simulink model "TPF_Control_Automatico_SLX"  (R2021a)
settings: Solver=ode4  StartTime=0.0  StopTime=30  FixedStep=1e-3  RelTol=1e-3
PreLoadFcn:
  | cuentas_pendulo_doble_final;
InitFcn:
  | cuentas_pendulo_doble_final;
values from neighbouring files (symbols this model uses):
  I0 = 0    [TPF_Control_Automatico.m]    (also in cuentas_pendulo_doble_final.m)
  I1 = m1_value*(((L1_value)^2)/12)    (= 0.0833333333333)    [TPF_Control_Automatico.m]    (also in cuentas_pendulo_doble_final.m; cuentas_prueba.m = 0.0104166666667)
  I2 = m2_value*(((L2_value)^2)/12)    (= 0.1875)    [TPF_Control_Automatico.m]    (also in cuentas_pendulo_doble_final.m; cuentas_prueba.m = 0.03515625)
  K = place(sys.A, sys.B, [-3 -2.5 -2.4 -2 -1.9 -1.8])    [TPF_Control_Automatico.m]    (also in cuentas_pendulo_doble.m = acker(A,B,[0.002,-0.001,-0.001,-0.001,-0.001,-0.001]); cuentas_pendulo_doble_final.m = place(sys.A, sys.B, [-4 -3.5 -3 -2.5 -2 -1.5]); cuentas_prueba.m = acker(sys.A, sys.B, [-3 -3 -2 -2]))
  KDisc = place(sysDisc.A, sysDisc.B, exp([-1.5 -1.6 -1.7 -2 -2.1 -2.2].*Ts))    [TPF_Control_Automatico.m]    (also in cuentas_pendulo_doble_final.m = place(sysDisc.A, sysDisc.B, exp([-3.5 -3 -2.5 -2 -1.5 -1].*T; cuentas_prueba.m = acker(sysDisc.A, sysDisc.B, exp([-2 -2 -1 -1].*Ts)))
  L = place((sys.A)',(sys.C)', [-3 -2.5 -2.4 -2 -1.9 -1.8].*10)'    [TPF_Control_Automatico.m]    (also in cuentas_pendulo_doble.m = [zeros(3,1); cuentas_pendulo_doble_final.m = place((sys.A)',(sys.C)', [-4 -3.5 -3 -2.5 -2 -1.5].*15)'; cuentas_prueba.m = place((sys.A)',(sys.C)', [-25 -20 -35 -30])')
  L1_value = 1    [TPF_Control_Automatico.m]    (also in cuentas_pendulo_doble.m = 0.5; cuentas_pendulo_doble_final.m; cuentas_prueba.m = 0.5)
  L2_value = 1.5    [TPF_Control_Automatico.m]    (also in cuentas_pendulo_doble.m = 0.75; cuentas_pendulo_doble_final.m; cuentas_prueba.m = 0.75)
  LDisc = place((sysDisc.A)',(sysDisc.C)', exp(([-1.5 -1.6 -1.7 -2 -2.1 -2.2].*20).*Ts))'    [TPF_Control_Automatico.m]    (also in cuentas_pendulo_doble_final.m = place((sysDisc.A)',(sysDisc.C)', exp(([-3.5 -3 -2.5 -2 -1.5 ; cuentas_prueba.m = place((sysDisc.A)',(sysDisc.C)', exp([-20 -15 -25 -30].*Ts)))
  m0_value = 5    [TPF_Control_Automatico.m]    (also in cuentas_pendulo_doble.m = 1.5; cuentas_pendulo_doble_final.m; cuentas_prueba.m = 1.5)
  m1_value = 1    [TPF_Control_Automatico.m]    (also in cuentas_pendulo_doble.m = 0.5; cuentas_pendulo_doble_final.m; cuentas_prueba.m = 0.5)
  m2_value = 1    [TPF_Control_Automatico.m]    (also in cuentas_pendulo_doble.m = 0.75; cuentas_pendulo_doble_final.m; cuentas_prueba.m = 0.75)
  s = tf('s')    [TPF_Control_Automatico.m]    (also in cuentas_pendulo_doble.m; cuentas_pendulo_doble_final.m; cuentas_prueba.m)
  sys = ss(A,B,C,D)    [TPF_Control_Automatico.m]    (also in cuentas_pendulo_doble_final.m; cuentas_prueba.m)
  sysDisc = c2d(sys, Ts, 'tustin')    [TPF_Control_Automatico.m]    (also in cuentas_pendulo_doble_final.m; cuentas_prueba.m)
  Ts = 0.03    [TPF_Control_Automatico.m]    (also in cuentas_pendulo_doble_final.m = 0.025; cuentas_prueba.m = 0.1)
undefined symbols (not defined in the file or in its folder): X, Y, Z
libraries: sm_lib x60, nesl_utility x30, eeGeneralControl x3
(part 1 of 2)
settings Model: Creator=Acer  LastModifiedBy=alan_

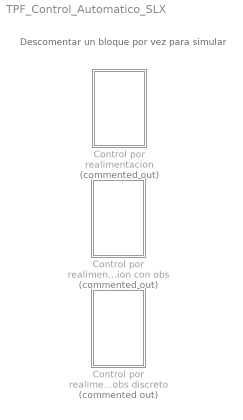
== system TPF_Control_Automatico_SLX ==
  note: Descomentar un bloque por vez para simular
  Control por realimentacion : Subsystem  Commented=on
  Control por realimentacion con obs : Subsystem  Commented=on
  Control por realimentacion con obs discreto : Subsystem  Commented=on

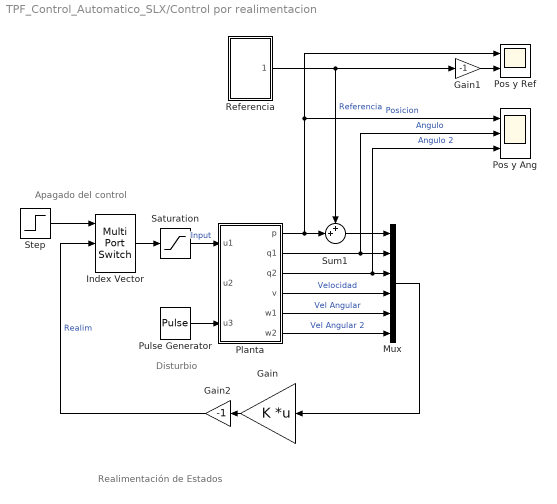
== system TPF_Control_Automatico_SLX/Control por realimentacion ==
  note: Disturbio
  note: Apagado del control
  note: Realimentación de Estados
  Gain : Gain  Gain=K  Multiplication=Matrix(K*u) (u vector)
  Gain1 : Gain  Gain=-1
  Gain2 : Gain  Gain=-1
  Index Vector : MultiPortSwitch  DataPortOrder=Zero-based contiguous  Inputs=2  zeroidx=on
  Mux : Mux  Inputs=6
  Planta : Subsystem  mask{carro_masa=m0_value, barra1_masa=m1_value, barra2_masa=m2_value, barra1_long=L1_value, barra2_long=L2_value}
      mask prompts: carro_masa "Masa del carro"; barra1_masa "Masa primera barra"; barra2_masa "Masa segunda barra"; barra1_long "Longitud primera barra"; barra2_long "Longitud segunda barra"
  Pos y Ang : Scope  NumInputPorts=3
  Pos y Ref : Scope  NumInputPorts=2
  Pulse Generator : DiscretePulseGenerator  PulseType=Time based  Amplitude=0.5  Period=100  PulseWidth=0.1  PhaseDelay=10
  Referencia : Subsystem
  Saturation : Saturate  UpperLimit=500  LowerLimit=-500
  Step : Step  Time=18  SampleTime=0
  Sum1 : Sum  Inputs=++|
  wires:
  Planta/2(q1) -> Mux/2, Pos y Ang/2  "Angulo"
  Gain/1 -> Gain2/1
  Referencia/1(Posición) -> Sum1/1, Gain1/1  "Referencia"
  Gain1/1 -> Pos y Ref/2
  Sum1/1 -> Mux/1
  Planta/3(q2) -> Pos y Ang/3, Mux/3  "Angulo 2"
  Planta/4(v) -> Mux/4  "Velocidad"
  Planta/5(w1) -> Mux/5  "Vel Angular"
  Planta/6(w2) -> Mux/6  "Vel Angular 2"
  Mux/1 -> Gain/1
  Saturation/1 -> Planta/1(u1)  "Input"
  Planta/1(p) -> Pos y Ref/1, Pos y Ang/1, Sum1/2  "Posicion"
  Pulse Generator/1 -> Planta/3(u3)
  Gain2/1 -> Index Vector/2  "Realim"
  Index Vector/1 -> Saturation/1
  Step/1 -> Index Vector/1

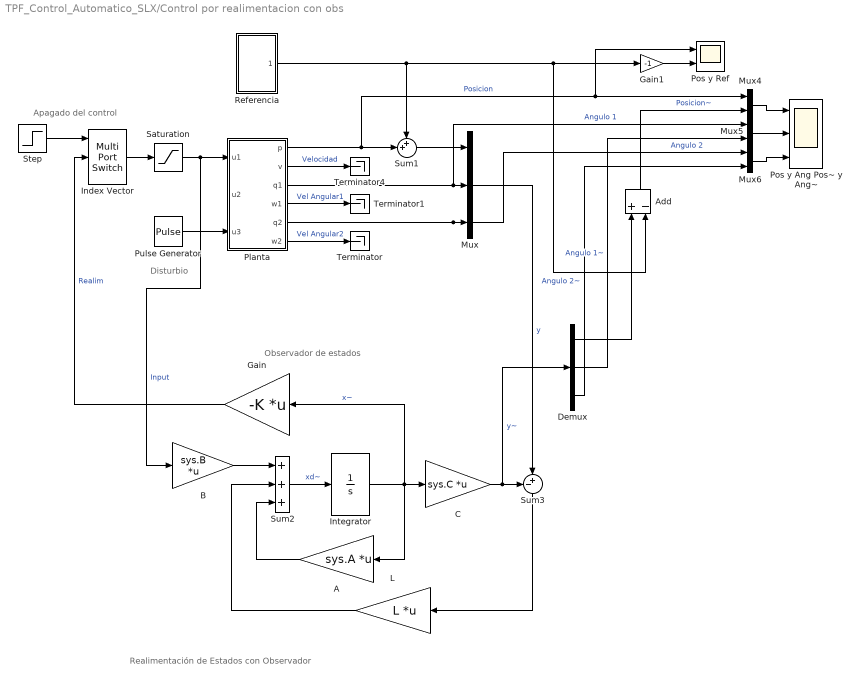
== system TPF_Control_Automatico_SLX/Control por realimentacion con obs ==
  note: Observador de estados
  note: Disturbio
  note: Realimentación de Estados con Observador
  note: Apagado del control
  A : Gain  Gain=sys.A  Multiplication=Matrix(K*u) (u vector)
  Add : Sum  Inputs=+-
  B : Gain  Gain=sys.B  Multiplication=Matrix(K*u) (u vector)
  C : Gain  Gain=sys.C  Multiplication=Matrix(K*u) (u vector)
  Demux : Demux  Outputs=3
  Gain : Gain  Gain=-K  Multiplication=Matrix(K*u) (u vector)
  Gain1 : Gain  Gain=-1
  Index Vector : MultiPortSwitch  DataPortOrder=Zero-based contiguous  Inputs=2  zeroidx=on
  Integrator : Integrator  InitialCondition=[0 0 0 0 0 0]
  L : Gain  Gain=L  Multiplication=Matrix(K*u) (u vector)
  Mux : Mux  Inputs=3
  Mux4 : Mux  Inputs=2
  Mux5 : Mux  Inputs=2
  Mux6 : Mux  Inputs=2
  Planta : Subsystem  mask{carro_masa=m0_value, barra1_masa=m1_value, barra2_masa=m2_value, barra1_long=L1_value, barra2_long=L2_value}
      mask prompts: carro_masa "Masa del carro"; barra1_masa "Masa primera barra"; barra2_masa "Masa segunda barra"; barra1_long "Longitud primera barra"; barra2_long "Longitud segunda barra"
  Pos y Ang Pos~ y Ang~ : Scope  NumInputPorts=3
  Pos y Ref : Scope  NumInputPorts=2
  Pulse Generator : DiscretePulseGenerator  PulseType=Time based  Amplitude=0.5  Period=100  PulseWidth=0.1  PhaseDelay=10
  Referencia : Subsystem
  Saturation : Saturate  UpperLimit=500  LowerLimit=-500
  Step : Step  Time=18  SampleTime=0
  Sum1 : Sum  Inputs=++|
  Sum2 : Sum  Inputs=+++
  Sum3 : Sum  Inputs=-+|
  Terminator : Terminator
  Terminator1 : Terminator
  Terminator4 : Terminator
  wires:
  Integrator/1 -> Gain/1, C/1, A/1  "x~"
  Sum2/1 -> Integrator/1  "xd~"
  A/1 -> Sum2/3
  B/1 -> Sum2/1
  Sum3/1 -> L/1
  L/1 -> Sum2/2
  C/1 -> Demux/1, Sum3/1  "y~"
  Mux/1 -> Sum3/2  "y"
  Sum1/1 -> Mux/1
  Referencia/1(Posición) -> Gain1/1, Add/2, Sum1/1
  Gain1/1 -> Pos y Ref/2
  Planta/1(p) -> Sum1/2, Pos y Ref/1, Mux4/1  "Posicion"
  Planta/3(q1) -> Mux5/1, Mux/2  "Angulo 1"
  Planta/6(w2) -> Terminator/1  "Vel Angular2"
  Planta/4(w1) -> Terminator1/1  "Vel Angular1"
  Planta/2(v) -> Terminator4/1  "Velocidad"
  Planta/5(q2) -> Mux6/1, Mux/3  "Angulo 2"
  Saturation/1 -> Planta/1(u1), B/1  "Input"
  Gain/1 -> Index Vector/2  "Realim"
  Step/1 -> Index Vector/1
  Index Vector/1 -> Saturation/1
  Pulse Generator/1 -> Planta/3(u3)
  Mux4/1 -> Pos y Ang Pos~ y Ang~/1
  Mux5/1 -> Pos y Ang Pos~ y Ang~/2
  Mux6/1 -> Pos y Ang Pos~ y Ang~/3
  Demux/2 -> Mux5/2  "Angulo 1~"
  Demux/3 -> Mux6/2  "Angulo 2~"
  Demux/1 -> Add/1
  Add/1 -> Mux4/2  "Posicion~"

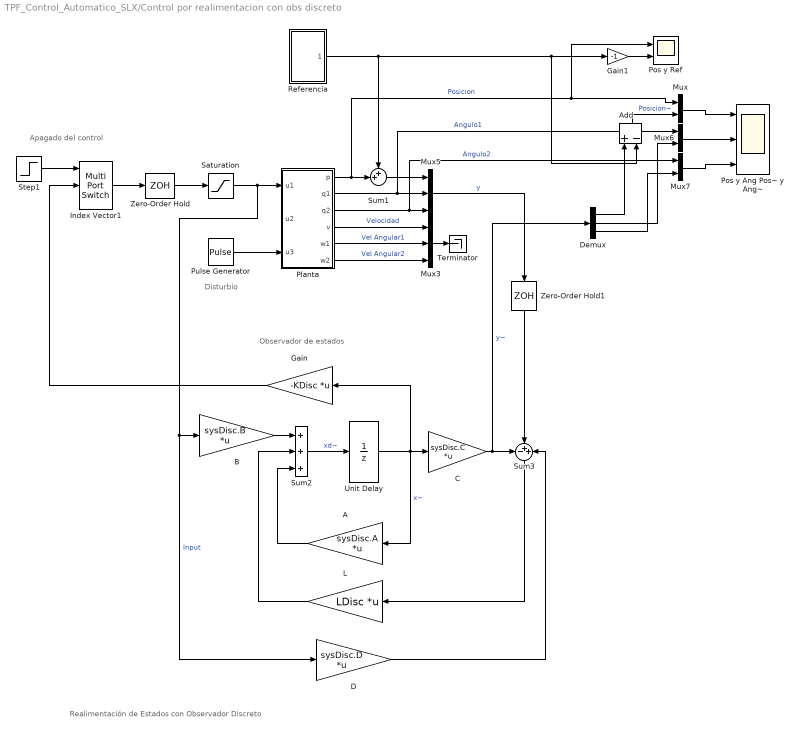
== system TPF_Control_Automatico_SLX/Control por realimentacion con obs discreto ==
  note: Observador de estados
  note: Disturbio
  note: Realimentación de Estados con Observador Discreto
  note: Apagado del control
  A : Gain  Gain=sysDisc.A  Multiplication=Matrix(K*u) (u vector)
  Add : Sum  Inputs=+-
  B : Gain  Gain=sysDisc.B  Multiplication=Matrix(K*u) (u vector)
  C : Gain  Gain=sysDisc.C  Multiplication=Matrix(K*u) (u vector)
  D : Gain  Gain=sysDisc.D  Multiplication=Matrix(K*u) (u vector)
  Demux : Demux  Outputs=3
  Gain : Gain  Gain=-KDisc  Multiplication=Matrix(K*u) (u vector)
  Gain1 : Gain  Gain=-1
  Index Vector1 : MultiPortSwitch  DataPortOrder=Zero-based contiguous  Inputs=2  zeroidx=on
  L : Gain  Gain=LDisc  Multiplication=Matrix(K*u) (u vector)
  Mux : Mux  Inputs=2
  Mux3 : Mux  Inputs=3
  Mux5 : Mux  Inputs=3
  Mux6 : Mux  Inputs=2
  Mux7 : Mux  Inputs=2
  Planta : Subsystem  mask{carro_masa=m0_value, barra1_masa=m1_value, barra2_masa=m2_value, barra1_long=L1_value, barra2_long=L2_value}
      mask prompts: carro_masa "Masa del carro"; barra1_masa "Masa primera barra"; barra2_masa "Masa segunda barra"; barra1_long "Longitud primera barra"; barra2_long "Longitud segunda barra"
  Pos y Ang Pos~ y Ang~ : Scope  NumInputPorts=3
  Pos y Ref : Scope  NumInputPorts=2
  Pulse Generator : DiscretePulseGenerator  PulseType=Time based  Amplitude=0.5  Period=100  PulseWidth=0.1  PhaseDelay=10
  Referencia : Subsystem
  Saturation : Saturate  UpperLimit=500  LowerLimit=-500
  Step1 : Step  Time=18  SampleTime=0
  Sum1 : Sum  Inputs=++|
  Sum2 : Sum  Inputs=+++
  Sum3 : Sum  Inputs=-++
  Terminator : Terminator
  Unit Delay : UnitDelay  InitialCondition=[0 0 0 0 0 0]  SampleTime=Ts  HasFrameUpgradeWarning=on
  Zero-Order Hold : ZeroOrderHold  SampleTime=Ts
  Zero-Order Hold1 : ZeroOrderHold  SampleTime=Ts
  wires:
  Sum2/1 -> Unit Delay/1  "xd~"
  A/1 -> Sum2/3
  B/1 -> Sum2/1
  Sum3/1 -> L/1
  L/1 -> Sum2/2
  D/1 -> Sum3/3
  Zero-Order Hold/1 -> Saturation/1
  Zero-Order Hold1/1 -> Sum3/2
  Planta/1(p) -> Mux/1, Pos y Ref/1, Sum1/2  "Posicion"
  Unit Delay/1 -> Gain/1, C/1, A/1  "x~"
  Referencia/1(Posición) -> Add/2, Gain1/1, Sum1/1
  Mux5/1 -> Zero-Order Hold1/1  "y"
  Gain1/1 -> Pos y Ref/2
  C/1 -> Demux/1, Sum3/1  "y~"
  Sum1/1 -> Mux5/1
  Planta/2(q1) -> Mux6/1, Mux5/2  "Angulo1"
  Planta/3(q2) -> Mux7/1, Mux5/3  "Angulo2"
  Planta/4(v) -> Mux3/1  "Velocidad"
  Planta/5(w1) -> Mux3/2  "Vel Angular1"
  Planta/6(w2) -> Mux3/3  "Vel Angular2"
  Mux3/1 -> Terminator/1
  Saturation/1 -> Planta/1(u1), B/1, D/1  "Input"
  Pulse Generator/1 -> Planta/3(u3)
  Step1/1 -> Index Vector1/1
  Index Vector1/1 -> Zero-Order Hold/1
  Gain/1 -> Index Vector1/2
  Mux/1 -> Pos y Ang Pos~ y Ang~/1
  Mux6/1 -> Pos y Ang Pos~ y Ang~/2
  Mux7/1 -> Pos y Ang Pos~ y Ang~/3
  Demux/2 -> Mux6/2
  Demux/3 -> Mux7/2
  Add/1 -> Mux/2  "Posicion~"
  Demux/1 -> Add/1

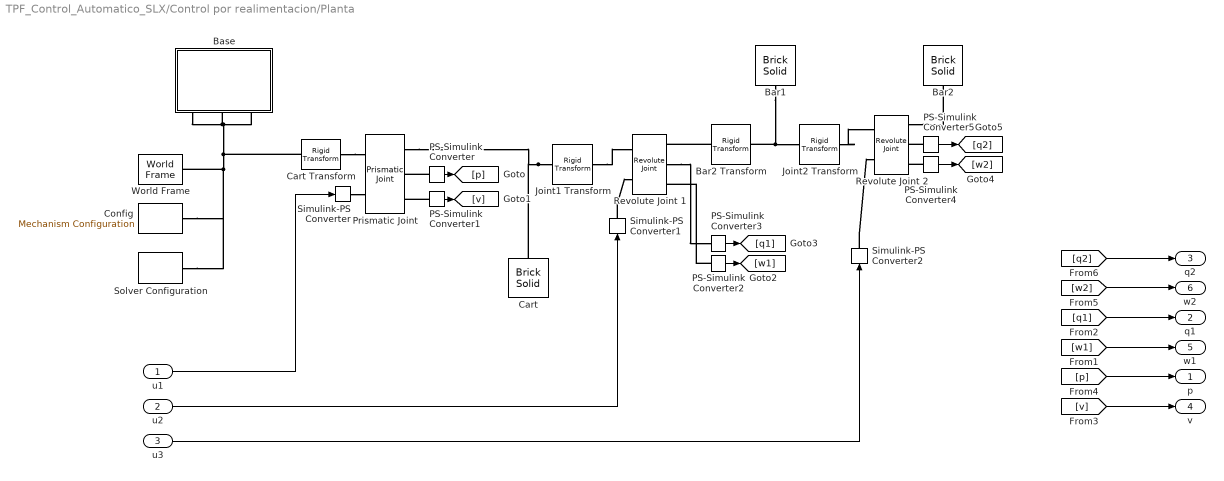
== system TPF_Control_Automatico_SLX/Control por realimentacion/Planta ==
  u1 : Inport
  u2 : Inport  Port=2
  u3 : Inport  Port=3
  Bar1 : sm_lib/Body Elements/Brick Solid  GraphicAmbientColor=[0.15 0.15 0.15 1.0]  BasedOnType=Mass  BrickDimensions=[barra1_long 0.1 0.1]  BrickDimensionUnits=m  CenterOfMass=[0 0 0]  CenterOfMassUnits=m  GraphicDiffuseColor=[0.8 0.0 0.0]  Density=1000  DensityUnits=kg/m^3  DoExposeReferenceFrame=off  GraphicEmissiveColor=[0.0 0.0 0.0 1.0]  ExportEntireGeometry=off  SerializedFrames=<Frames><Frame><Id>Frame1</Id><Value><Name>F1</Name><Origin><Source>GeometricFeature</Source><FeatureName>+x surface</FeatureName></Origin><PrimaryAxis><DefinedDirection>+Z</DefinedDirection><Source>ReferenceFrame</Source><SourceDirection>+Z</SourceDirection><FeatureName></FeatureName></PrimaryAxis><SecondaryAxis><DefinedDirection>+X</DefinedDirection><Source>ReferenceFrame</Source><SourceDirection>+X</SourceDirection><FeatureName></FeatureName></SecondaryAxis></Value></Frame></Frames>  MarkerShape=Sphere  MarkerSize=10  GraphicType=FromGeometry  InertiaType=Custom  Mass=barra1_masa  MassUnits=kg  MomentsOfInertia=[I0 I1 I1]  MomentsOfInertiaUnits=kg*m^2  GraphicOpacity=1.0  ProductsOfInertia=[0 0 0]  ProductsOfInertiaUnits=kg*m^2  GraphicShininess=75  GraphicSpecularColor=[0.5 0.5 0.5 1.0]  GraphicVisPropType=SimpleVisualProperties
  Bar2 : sm_lib/Body Elements/Brick Solid  GraphicAmbientColor=[0.15 0.15 0.15 1.0]  BasedOnType=Mass  BrickDimensions=[barra2_long 0.1 0.1]  BrickDimensionUnits=m  CenterOfMass=[0 0 0]  CenterOfMassUnits=m  GraphicDiffuseColor=[0.0 0.2 0.8]  Density=1000  DensityUnits=kg/m^3  DoExposeReferenceFrame=off  GraphicEmissiveColor=[0.0 0.0 0.0 1.0]  ExportEntireGeometry=off  SerializedFrames=<Frames><Frame><Id>Frame1</Id><Value><Name>F1</Name><Origin><Source>GeometricFeature</Source><FeatureName>+x surface</FeatureName></Origin><PrimaryAxis><DefinedDirection>+Z</DefinedDirection><Source>ReferenceFrame</Source><SourceDirection>+Z</SourceDirection><FeatureName></FeatureName></PrimaryAxis><SecondaryAxis><DefinedDirection>+X</DefinedDirection><Source>ReferenceFrame</Source><SourceDirection>+X</SourceDirection><FeatureName></FeatureName></SecondaryAxis></Value></Frame></Frames>  MarkerShape=Sphere  MarkerSize=10  GraphicType=FromGeometry  InertiaType=Custom  Mass=barra2_masa  MassUnits=kg  MomentsOfInertia=[I0 I2 I2]  MomentsOfInertiaUnits=kg*m^2  GraphicOpacity=1.0  ProductsOfInertia=[0 0 0]  ProductsOfInertiaUnits=kg*m^2  GraphicShininess=75  GraphicSpecularColor=[0.5 0.5 0.5 1.0]  GraphicVisPropType=SimpleVisualProperties
  Bar2 Transform : sm_lib/Frames and Transforms/Rigid Transform  TranslationMethod=StandardAxis  TranslationStandardOffset=0  TranslationLengthUnit=m  TranslationStandardAxis=+Z  TranslationCartesianOffset=[0 0 0]  TranslationROffset=0  TranslationROffsetUnits=m  TranslationZOffset=0  TranslationZOffsetUnits=m  TranslationThetaOffset=0  TranslationThetaOffsetUnits=deg  RotationMethod=RotationSequence  RotationAngleUnits=deg  RotationStandardAxis=+Z  RotationAngle=0.0  RotationArbitraryAxis=[0 0 1]  FollAlignAxisA=+X  BaseAlignAxisA=+Y  FollAlignAxisB=+Y  BaseAlignAxisB=+Z  RotationSequenceAxes=FollowerAxes  RotationSequence=XYZ  RotationSequenceAngles=[0 0 0]  RotationSequenceAnglesUnits=deg  RotationMatrix=[1 0 0; 0 1 0; 0 0 1]
  Base : Subsystem
      settings: PortSchema="{\"entries\":[{\"content\":{\"sides\":[{\"content\":{\"connectorIds\":[]},\"type\":\"ConnectorPlacement.EquallySpacedRectSide\",\"uuid\":\"4332d69e-9bfe-4e89-a576-e2f6915cd745\"},{\"content\":{\"connectorIds\":[],\"side\":\"RIGHT\"},\"type\":\"ConnectorPlacement.EquallySpacedRectSide\",\"uuid\":\"1cc8b419-5de1-497b-b007-7cad9f99b098\"},{\"content\":{\"connectorIds\":[],\"side\":\"TOP\"},\"type\":\"ConnectorPlacement.EquallySpacedRectSide\",\"uuid\":\"21186588-641c-464a-a5f8-9ec189ea03bb\"},{\"content\":{\"connectorIds\":[\"RConn1\",\"RConn2\",\"RConn3\"],\"side\":\"BOTTOM\"},\"type\":\"ConnectorPlacement.EquallySpacedRectSide\",\"uuid\":\"3296c54c-d68e-452d-9e4e-a58ba512af2d\"}]},\"type\":\"ConnectorPlacement.EquallySpacedConnector\",\"uuid\":\"cf495630-4c35-4c65-b481-9d90798c8966\"}],\"packageUris\":[\"http://schema.mathworks.com/mf0/Connector/R2020b\"],\"version\":\"1.0\"}"
  Cart : sm_lib/Body Elements/Brick Solid  GraphicAmbientColor=[0.15 0.15 0.15 1.0]  BasedOnType=Mass  BrickDimensions=[0.05 1 1.5]  BrickDimensionUnits=m  CenterOfMass=[0 0 0]  CenterOfMassUnits=m  GraphicDiffuseColor=[0.2 0.2 0.2]  Density=1000  DensityUnits=kg/m^3  DoExposeReferenceFrame=on  GraphicEmissiveColor=[0.0 0.0 0.0 1.0]  ExportEntireGeometry=off  SerializedFrames=<Frames/>  MarkerShape=Sphere  MarkerSize=10  GraphicType=FromGeometry  InertiaType=Custom  Mass=carro_masa  MassUnits=kg  MomentsOfInertia=[1 1 1]  MomentsOfInertiaUnits=kg*m^2  GraphicOpacity=1.0  ProductsOfInertia=[0 0 0]  ProductsOfInertiaUnits=kg*m^2  GraphicShininess=75  GraphicSpecularColor=[0.5 0.5 0.5 1.0]  GraphicVisPropType=SimpleVisualProperties
  Cart Transform : sm_lib/Frames and Transforms/Rigid Transform  TranslationMethod=StandardAxis  TranslationStandardOffset=0  TranslationLengthUnit=m  TranslationStandardAxis=+Z  TranslationCartesianOffset=[0 0 0]  TranslationROffset=0  TranslationROffsetUnits=m  TranslationZOffset=0  TranslationZOffsetUnits=m  TranslationThetaOffset=0  TranslationThetaOffsetUnits=deg  RotationMethod=RotationSequence  RotationAngleUnits=deg  RotationStandardAxis=+Z  RotationAngle=0.0  RotationArbitraryAxis=[0 0 1]  FollAlignAxisA=+X  BaseAlignAxisA=+Y  FollAlignAxisB=+Y  BaseAlignAxisB=+Z  RotationSequenceAxes=FollowerAxes  RotationSequence=XYZ  RotationSequenceAngles=[0 90 0]  RotationSequenceAnglesUnits=deg  RotationMatrix=[1 0 0; 0 1 0; 0 0 1]
  Config : sm_lib/Utilities/Mechanism Configuration  UniformGravity=Constant  GravityVector=[0 0 -9.8]  GravityVectorUnits=m/s^2  GravityUnits=m/s^2  LinearizationDelta=0.0001  JointModeTransitionNonlinearIterations=2
  Joint1 Transform : sm_lib/Frames and Transforms/Rigid Transform  TranslationMethod=StandardAxis  TranslationStandardOffset=0  TranslationLengthUnit=m  TranslationStandardAxis=+X  TranslationCartesianOffset=[0 0 0]  TranslationROffset=0  TranslationROffsetUnits=m  TranslationZOffset=0  TranslationZOffsetUnits=m  TranslationThetaOffset=0  TranslationThetaOffsetUnits=deg  RotationMethod=RotationSequence  RotationAngleUnits=deg  RotationStandardAxis=+Z  RotationAngle=0.0  RotationArbitraryAxis=[0 0 1]  FollAlignAxisA=+X  BaseAlignAxisA=+Y  FollAlignAxisB=+Y  BaseAlignAxisB=+Z  RotationSequenceAxes=FollowerAxes  RotationSequence=XYZ  RotationSequenceAngles=[270 0 0]  RotationSequenceAnglesUnits=deg  RotationMatrix=[1 0 0; 0 1 0; 0 0 1]
  Joint2 Transform : sm_lib/Frames and Transforms/Rigid Transform  TranslationMethod=StandardAxis  TranslationStandardOffset=barra1_long  TranslationLengthUnit=m  TranslationStandardAxis=-X  TranslationCartesianOffset=[0 0 0]  TranslationROffset=0  TranslationROffsetUnits=m  TranslationZOffset=0  TranslationZOffsetUnits=m  TranslationThetaOffset=0  TranslationThetaOffsetUnits=deg  RotationMethod=RotationSequence  RotationAngleUnits=deg  RotationStandardAxis=+Z  RotationAngle=0.0  RotationArbitraryAxis=[0 0 1]  FollAlignAxisA=+X  BaseAlignAxisA=+Y  FollAlignAxisB=+Y  BaseAlignAxisB=+Z  RotationSequenceAxes=FollowerAxes  RotationSequence=XYZ  RotationSequenceAngles=[0 0 0]  RotationSequenceAnglesUnits=deg  RotationMatrix=[1 0 0; 0 1 0; 0 0 1]
  PS-Simulink Converter{,1..5} (6 alike) : nesl_utility/PS-Simulink Converter  PhysicalDomain=network_engine_domain  SubClassName=ps_output  LeftPortType=input  RightPortType=output  PseudoPeriodic=off  Frequencies=[]  Unit=inherit  AffineConversion=off
      settings: SourceProductBaseCode=PW,SS
  Prismatic Joint : sm_lib/Joints/Prismatic Joint  JointMode=Normal  SenseConstraintForce=off  SenseConstraintForceX=off  SenseConstraintForceY=off  SenseConstraintForceZ=off  SenseConstraintTorque=off  SenseConstraintTorqueX=off  SenseConstraintTorqueY=off  SenseConstraintTorqueZ=off  SenseTotalForce=off  SenseTotalForceX=off  SenseTotalForceY=off  SenseTotalForceZ=off  SenseTotalTorque=off  SenseTotalTorqueX=off  SenseTotalTorqueY=off  SenseTotalTorqueZ=off  CompositeWrenchDir=FollowerOnBase  CompositeWrenchFrame=BaseFrame  EquilibriumPosition=0  EquilibriumPositionUnits=m  SpringStiffness=0  SpringStiffnessUnits=N/m  DampingCoefficient=F0  DampingCoefficientUnits=N/(m/s)  TorqueActuationMode=InputTorque  MotionActuationMode=ComputedMotion  SensePosition=on  SenseVelocity=on  SenseAcceleration=off  SenseTorqueForce=off  SenseLowerLimitTorqueForce=off  SenseUpperLimitTorqueForce=off  LowerLimitSpecify=on  LowerLimitBound=-10  LowerLimitBoundUnits=m  LowerLimitStiffness=1e6  LowerLimitStiffnessUnits=N/m  LowerLimitDamping=1e3  LowerLimitDampingUnits=N/(m/s)  LowerLimitTransitionRegionWidth=1e-4  LowerLimitTransitionRegionWidthUnits=m  UpperLimitSpecify=on  UpperLimitBound=10  UpperLimitBoundUnits=m  UpperLimitStiffness=1e6  UpperLimitStiffnessUnits=N/m  UpperLimitDamping=1e3  UpperLimitDampingUnits=N/(m/s)  UpperLimitTransitionRegionWidth=1e-4  UpperLimitTransitionRegionWidthUnits=m  PositionTargetSpecify=off  PositionTargetPriority=High  PositionTargetValue=0  PositionTargetValueUnits=m  VelocityTargetSpecify=off  VelocityTargetPriority=High  VelocityTargetValue=0  VelocityTargetValueUnits=m/s
  Revolute Joint 1 : sm_lib/Joints/Revolute Joint  JointMode=Normal  SenseConstraintForce=off  SenseConstraintForceX=off  SenseConstraintForceY=off  SenseConstraintForceZ=off  SenseConstraintTorque=off  SenseConstraintTorqueX=off  SenseConstraintTorqueY=off  SenseConstraintTorqueZ=off  SenseTotalForce=off  SenseTotalForceX=off  SenseTotalForceY=off  SenseTotalForceZ=off  SenseTotalTorque=off  SenseTotalTorqueX=off  SenseTotalTorqueY=off  SenseTotalTorqueZ=off  CompositeWrenchDir=FollowerOnBase  CompositeWrenchFrame=BaseFrame  EquilibriumPosition=0  EquilibriumPositionUnits=deg  SpringStiffness=0  SpringStiffnessUnits=N*m/deg  DampingCoefficient=F1  DampingCoefficientUnits=N*m/(deg/s)  TorqueActuationMode=InputTorque  MotionActuationMode=ComputedMotion  SensePosition=on  SenseVelocity=on  SenseAcceleration=off  SenseTorqueForce=off  SenseLowerLimitTorqueForce=off  SenseUpperLimitTorqueForce=off  LowerLimitSpecify=off  LowerLimitBound=-90  LowerLimitBoundUnits=deg  LowerLimitStiffness=1e4  LowerLimitStiffnessUnits=N*m/deg  LowerLimitDamping=10  LowerLimitDampingUnits=N*m/(deg/s)  LowerLimitTransitionRegionWidth=0.1  LowerLimitTransitionRegionWidthUnits=deg  UpperLimitSpecify=off  UpperLimitBound=90  UpperLimitBoundUnits=deg  UpperLimitStiffness=1e4  UpperLimitStiffnessUnits=N*m/deg  UpperLimitDamping=10  UpperLimitDampingUnits=N*m/(deg/s)  UpperLimitTransitionRegionWidth=0.1  UpperLimitTransitionRegionWidthUnits=deg  PositionTargetSpecify=off  PositionTargetPriority=Low  PositionTargetValue=0.001  PositionTargetValueUnits=deg  VelocityTargetSpecify=off  VelocityTargetPriority=High  VelocityTargetValue=0  VelocityTargetValueUnits=deg/s
  Revolute Joint 2 : sm_lib/Joints/Revolute Joint  JointMode=Normal  SenseConstraintForce=off  SenseConstraintForceX=off  SenseConstraintForceY=off  SenseConstraintForceZ=off  SenseConstraintTorque=off  SenseConstraintTorqueX=off  SenseConstraintTorqueY=off  SenseConstraintTorqueZ=off  SenseTotalForce=off  SenseTotalForceX=off  SenseTotalForceY=off  SenseTotalForceZ=off  SenseTotalTorque=off  SenseTotalTorqueX=off  SenseTotalTorqueY=off  SenseTotalTorqueZ=off  CompositeWrenchDir=FollowerOnBase  CompositeWrenchFrame=BaseFrame  EquilibriumPosition=0  EquilibriumPositionUnits=deg  SpringStiffness=0  SpringStiffnessUnits=N*m/deg  DampingCoefficient=F2  DampingCoefficientUnits=N*m/(deg/s)  TorqueActuationMode=InputTorque  MotionActuationMode=ComputedMotion  SensePosition=on  SenseVelocity=on  SenseAcceleration=off  SenseTorqueForce=off  SenseLowerLimitTorqueForce=off  SenseUpperLimitTorqueForce=off  LowerLimitSpecify=off  LowerLimitBound=-90  LowerLimitBoundUnits=deg  LowerLimitStiffness=1e4  LowerLimitStiffnessUnits=N*m/deg  LowerLimitDamping=10  LowerLimitDampingUnits=N*m/(deg/s)  LowerLimitTransitionRegionWidth=0.1  LowerLimitTransitionRegionWidthUnits=deg  UpperLimitSpecify=off  UpperLimitBound=90  UpperLimitBoundUnits=deg  UpperLimitStiffness=1e4  UpperLimitStiffnessUnits=N*m/deg  UpperLimitDamping=10  UpperLimitDampingUnits=N*m/(deg/s)  UpperLimitTransitionRegionWidth=0.1  UpperLimitTransitionRegionWidthUnits=deg  PositionTargetSpecify=off  PositionTargetPriority=Low  PositionTargetValue=0.001  PositionTargetValueUnits=deg  VelocityTargetSpecify=off  VelocityTargetPriority=High  VelocityTargetValue=0  VelocityTargetValueUnits=deg/s
  Simulink-PS Converter : nesl_utility/Simulink-PS Converter  PhysicalDomain=network_engine_domain  SubClassName=ps_input  LeftPortType=input  RightPortType=output  PseudoPeriodic=off  Frequencies=[]  NoiseDistribution=none  NoiseParameters=[]  Unit=1  AffineConversion=off  FilteringAndDerivatives=provide  SimscapeFilterOrder=1  InputFilterTimeConstant=0.001  UdotUserProvided=0
      settings: SourceProductBaseCode=PW,SS
  Simulink-PS Converter1 : nesl_utility/Simulink-PS Converter  PhysicalDomain=network_engine_domain  SubClassName=ps_input  LeftPortType=input  RightPortType=output  PseudoPeriodic=off  Frequencies=[]  NoiseDistribution=none  NoiseParameters=[]  Unit=1  AffineConversion=off  FilteringAndDerivatives=provide  SimscapeFilterOrder=1  InputFilterTimeConstant=0.001  UdotUserProvided=0
      settings: SourceProductBaseCode=PW,SS
  Simulink-PS Converter2 : nesl_utility/Simulink-PS Converter  PhysicalDomain=network_engine_domain  SubClassName=ps_input  LeftPortType=input  RightPortType=output  PseudoPeriodic=off  Frequencies=[]  NoiseDistribution=none  NoiseParameters=[]  Unit=1  AffineConversion=off  FilteringAndDerivatives=provide  SimscapeFilterOrder=1  InputFilterTimeConstant=0.001  UdotUserProvided=0
      settings: SourceProductBaseCode=PW,SS
  Solver Configuration : nesl_utility/Solver Configuration  PhysicalDomain=network_engine_domain  SubClassName=solver  LeftPortType=input  RightPortType=generic  Tones=[]  Harmonics=[]  SimulateNoise=off  Profile=off  UseLocalSampling=off  EnableSwitchedLinearOptims=on  FrequencyDomain=off  UseCCode=off  RelTol=0.001  AbsTol=1e-06  MinStep=1e-09  ToWorkspace=off  RevertToSquareIcSolve=off  NumHomotopyIterations=100  PhasorMode=off  PhasorModeNumHarmonics=1  DoDC=off  ResidualTolerance=1e-09  UseLocalSolver=off  LocalSolverChoice=NE_BACKWARD_EULER_ADVANCER  LocalSolverSampleTime=0.001  DoFixedCost=off  MaxNonlinIter=3  MaxModeIter=2  ComputeImpulses=off  ImpulseIterations=2  LinearAlgebra=auto  EquationFormulation=NE_TIME_EF  DelaysMemoryBudget=1024  AutomaticFiltering=on  FilteringTimeConstant=0.001  PartitionStorageMethod=AS_NEEDED  PartitionMemoryBudget=1024  PartitionMethod=ROBUST
      settings: SourceProductBaseCode=PW,SS
  World Frame : sm_lib/Frames and Transforms/World Frame
  p : Outport
  q1 : Outport  Port=2
  q2 : Outport  Port=3
  v : Outport  Port=4
  w1 : Outport  Port=5
  w2 : Outport  Port=6
  wires:
  PS-Simulink Converter/1 -> [p]
  PS-Simulink Converter3/1 -> [q1]
  [q1] -> q1/1
  [p] -> p/1
  PS-Simulink Converter1/1 -> [v]
  PS-Simulink Converter2/1 -> [w1]
  [w1] -> w1/1
  [v] -> v/1
  u1/1 -> Simulink-PS Converter/1
  PS-Simulink Converter5/1 -> [q2]
  PS-Simulink Converter4/1 -> [w2]
  [w2] -> w2/1
  [q2] -> q2/1
  u2/1 -> Simulink-PS Converter1/1
  u3/1 -> Simulink-PS Converter2/1
  connections:
  PS-Simulink Converter1/LConn1 -- Prismatic Joint/RConn3
  Bar1/LConn1 -- Joint2 Transform/LConn1 -- Bar2 Transform/RConn1
  Bar2 Transform/LConn1 -- Revolute Joint 1/RConn1
  Base/RConn1 -- Base/RConn3 -- Cart Transform/LConn1 -- Config/RConn1 -- Solver Configuration/RConn1 -- World Frame/RConn1 -- Base/RConn2
  Cart Transform/RConn1 -- Prismatic Joint/LConn1
  PS-Simulink Converter/LConn1 -- Prismatic Joint/RConn2
  Simulink-PS Converter/RConn1 -- Prismatic Joint/LConn2
  PS-Simulink Converter2/LConn1 -- Revolute Joint 1/RConn3
  Joint1 Transform/RConn1 -- Revolute Joint 1/LConn1
  Revolute Joint 1/RConn2 -- PS-Simulink Converter3/LConn1
  Joint1 Transform/LConn1 -- Prismatic Joint/RConn1 -- Cart/RConn1
  PS-Simulink Converter4/LConn1 -- Revolute Joint 2/RConn3
  PS-Simulink Converter5/LConn1 -- Revolute Joint 2/RConn2
  Revolute Joint 2/RConn1 -- Bar2/LConn1
  Joint2 Transform/RConn1 -- Revolute Joint 2/LConn1
  Simulink-PS Converter1/RConn1 -- Revolute Joint 1/LConn2
  Simulink-PS Converter2/RConn1 -- Revolute Joint 2/LConn2

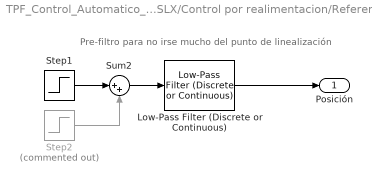
== system TPF_Control_Automatico_SLX/Control por realimentacion/Referencia ==
  note: Pre-filtro para no irse mucho del punto de linealización
  Low-Pass Filter (Discrete or Continuous) : eeGeneralControl/Low-Pass Filter (Discrete or Continuous)  K=1  T=1  B=inf  A=-inf  init_option=Inherited from block input  x0=0  Ts=-1
  Step1 : Step  After=4  SampleTime=0
  Step2 : Step  Commented=on  Time=8  After=-8  SampleTime=0
  Sum2 : Sum  Inputs=|++
  Posición : Outport
  wires:
  Step2/1 -> Sum2/2
  Sum2/1 -> Low-Pass Filter (Discrete or Continuous)/1
  Low-Pass Filter (Discrete or Continuous)/1 -> Posición/1
  Step1/1 -> Sum2/1

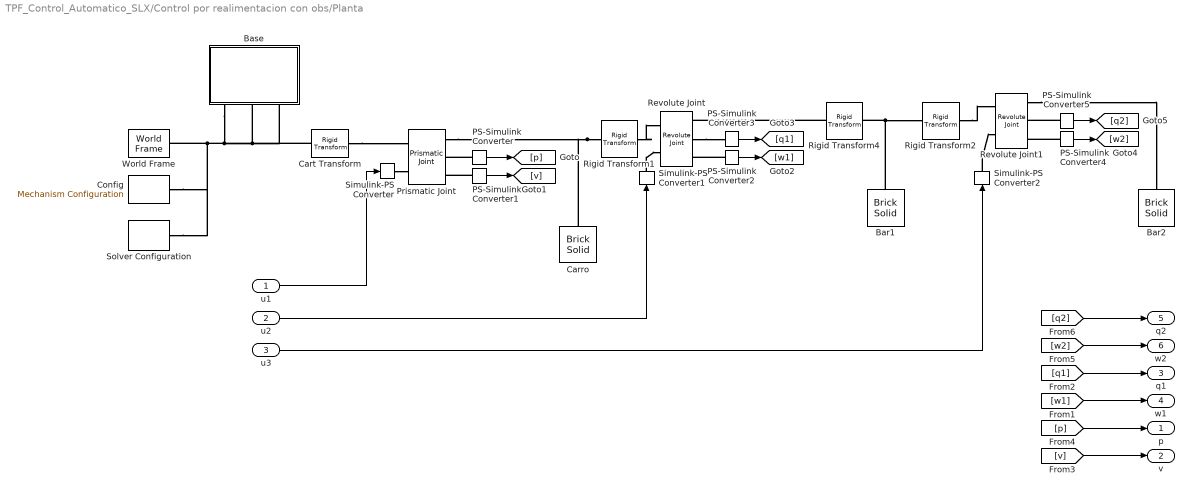
== system TPF_Control_Automatico_SLX/Control por realimentacion con obs/Planta ==
  u1 : Inport
  u2 : Inport  Port=2
  u3 : Inport  Port=3
  Bar1 : sm_lib/Body Elements/Brick Solid  GraphicAmbientColor=[0.15 0.15 0.15 1.0]  BasedOnType=Mass  BrickDimensions=[barra1_long 0.1 0.1]  BrickDimensionUnits=m  CenterOfMass=[0 0 0]  CenterOfMassUnits=m  GraphicDiffuseColor=[0.8 0.0 0.0]  Density=1000  DensityUnits=kg/m^3  DoExposeReferenceFrame=off  GraphicEmissiveColor=[0.0 0.0 0.0 1.0]  ExportEntireGeometry=off  SerializedFrames=<Frames><Frame><Id>Frame1</Id><Value><Name>F1</Name><Origin><Source>GeometricFeature</Source><FeatureName>+x surface</FeatureName></Origin><PrimaryAxis><DefinedDirection>+Z</DefinedDirection><Source>ReferenceFrame</Source><SourceDirection>+Z</SourceDirection><FeatureName></FeatureName></PrimaryAxis><SecondaryAxis><DefinedDirection>+X</DefinedDirection><Source>ReferenceFrame</Source><SourceDirection>+X</SourceDirection><FeatureName></FeatureName></SecondaryAxis></Value></Frame></Frames>  MarkerShape=Sphere  MarkerSize=10  GraphicType=FromGeometry  InertiaType=Custom  Mass=barra1_masa  MassUnits=kg  MomentsOfInertia=[I0 I1 I1]  MomentsOfInertiaUnits=kg*m^2  GraphicOpacity=1.0  ProductsOfInertia=[0 0 0]  ProductsOfInertiaUnits=kg*m^2  GraphicShininess=75  GraphicSpecularColor=[0.5 0.5 0.5 1.0]  GraphicVisPropType=SimpleVisualProperties
  Bar2 : sm_lib/Body Elements/Brick Solid  GraphicAmbientColor=[0.15 0.15 0.15 1.0]  BasedOnType=Mass  BrickDimensions=[barra2_long 0.1 0.1]  BrickDimensionUnits=m  CenterOfMass=[0 0 0]  CenterOfMassUnits=m  GraphicDiffuseColor=[0.0 0.2 0.8]  Density=1000  DensityUnits=kg/m^3  DoExposeReferenceFrame=off  GraphicEmissiveColor=[0.0 0.0 0.0 1.0]  ExportEntireGeometry=off  SerializedFrames=<Frames><Frame><Id>Frame1</Id><Value><Name>F1</Name><Origin><Source>GeometricFeature</Source><FeatureName>+x surface</FeatureName></Origin><PrimaryAxis><DefinedDirection>+Z</DefinedDirection><Source>ReferenceFrame</Source><SourceDirection>+Z</SourceDirection><FeatureName></FeatureName></PrimaryAxis><SecondaryAxis><DefinedDirection>+X</DefinedDirection><Source>ReferenceFrame</Source><SourceDirection>+X</SourceDirection><FeatureName></FeatureName></SecondaryAxis></Value></Frame></Frames>  MarkerShape=Sphere  MarkerSize=10  GraphicType=FromGeometry  InertiaType=Custom  Mass=barra2_masa  MassUnits=kg  MomentsOfInertia=[I0 I2 I2]  MomentsOfInertiaUnits=kg*m^2  GraphicOpacity=1.0  ProductsOfInertia=[0 0 0]  ProductsOfInertiaUnits=kg*m^2  GraphicShininess=75  GraphicSpecularColor=[0.5 0.5 0.5 1.0]  GraphicVisPropType=SimpleVisualProperties
  Base : Subsystem
      settings: PortSchema="{\"entries\":[{\"content\":{\"sides\":[{\"content\":{\"connectorIds\":[]},\"type\":\"ConnectorPlacement.EquallySpacedRectSide\",\"uuid\":\"4332d69e-9bfe-4e89-a576-e2f6915cd745\"},{\"content\":{\"connectorIds\":[],\"side\":\"RIGHT\"},\"type\":\"ConnectorPlacement.EquallySpacedRectSide\",\"uuid\":\"1cc8b419-5de1-497b-b007-7cad9f99b098\"},{\"content\":{\"connectorIds\":[],\"side\":\"TOP\"},\"type\":\"ConnectorPlacement.EquallySpacedRectSide\",\"uuid\":\"21186588-641c-464a-a5f8-9ec189ea03bb\"},{\"content\":{\"connectorIds\":[\"RConn1\",\"RConn2\",\"RConn3\"],\"side\":\"BOTTOM\"},\"type\":\"ConnectorPlacement.EquallySpacedRectSide\",\"uuid\":\"3296c54c-d68e-452d-9e4e-a58ba512af2d\"}]},\"type\":\"ConnectorPlacement.EquallySpacedConnector\",\"uuid\":\"cf495630-4c35-4c65-b481-9d90798c8966\"}],\"packageUris\":[\"http://schema.mathworks.com/mf0/Connector/R2020b\"],\"version\":\"1.0\"}"
  Carro : sm_lib/Body Elements/Brick Solid  GraphicAmbientColor=[0.15 0.15 0.15 1.0]  BasedOnType=Mass  BrickDimensions=[0.05 1 1.5]  BrickDimensionUnits=m  CenterOfMass=[0 0 0]  CenterOfMassUnits=m  GraphicDiffuseColor=[0.2 0.2 0.2]  Density=1000  DensityUnits=kg/m^3  DoExposeReferenceFrame=on  GraphicEmissiveColor=[0.0 0.0 0.0 1.0]  ExportEntireGeometry=off  SerializedFrames=<Frames/>  MarkerShape=Sphere  MarkerSize=10  GraphicType=FromGeometry  InertiaType=Custom  Mass=carro_masa  MassUnits=kg  MomentsOfInertia=[1 1 1]  MomentsOfInertiaUnits=kg*m^2  GraphicOpacity=1.0  ProductsOfInertia=[0 0 0]  ProductsOfInertiaUnits=kg*m^2  GraphicShininess=75  GraphicSpecularColor=[0.5 0.5 0.5 1.0]  GraphicVisPropType=SimpleVisualProperties
  Cart Transform : sm_lib/Frames and Transforms/Rigid Transform  TranslationMethod=StandardAxis  TranslationStandardOffset=0  TranslationLengthUnit=m  TranslationStandardAxis=+Z  TranslationCartesianOffset=[0 0 0]  TranslationROffset=0  TranslationROffsetUnits=m  TranslationZOffset=0  TranslationZOffsetUnits=m  TranslationThetaOffset=0  TranslationThetaOffsetUnits=deg  RotationMethod=RotationSequence  RotationAngleUnits=deg  RotationStandardAxis=+Z  RotationAngle=0.0  RotationArbitraryAxis=[0 0 1]  FollAlignAxisA=+X  BaseAlignAxisA=+Y  FollAlignAxisB=+Y  BaseAlignAxisB=+Z  RotationSequenceAxes=FollowerAxes  RotationSequence=XYZ  RotationSequenceAngles=[0 90 0]  RotationSequenceAnglesUnits=deg  RotationMatrix=[1 0 0; 0 1 0; 0 0 1]
  Config : sm_lib/Utilities/Mechanism Configuration  UniformGravity=Constant  GravityVector=[0 0 -9.8]  GravityVectorUnits=m/s^2  GravityUnits=m/s^2  LinearizationDelta=0.0001  JointModeTransitionNonlinearIterations=2
  PS-Simulink Converter{,1..5} (6 alike) : nesl_utility/PS-Simulink Converter  PhysicalDomain=network_engine_domain  SubClassName=ps_output  LeftPortType=input  RightPortType=output  PseudoPeriodic=off  Frequencies=[]  Unit=inherit  AffineConversion=off
      settings: SourceProductBaseCode=PW,SS
  Prismatic Joint : sm_lib/Joints/Prismatic Joint  JointMode=Normal  SenseConstraintForce=off  SenseConstraintForceX=off  SenseConstraintForceY=off  SenseConstraintForceZ=off  SenseConstraintTorque=off  SenseConstraintTorqueX=off  SenseConstraintTorqueY=off  SenseConstraintTorqueZ=off  SenseTotalForce=off  SenseTotalForceX=off  SenseTotalForceY=off  SenseTotalForceZ=off  SenseTotalTorque=off  SenseTotalTorqueX=off  SenseTotalTorqueY=off  SenseTotalTorqueZ=off  CompositeWrenchDir=FollowerOnBase  CompositeWrenchFrame=BaseFrame  EquilibriumPosition=0  EquilibriumPositionUnits=m  SpringStiffness=0  SpringStiffnessUnits=N/m  DampingCoefficient=F0  DampingCoefficientUnits=N/(m/s)  TorqueActuationMode=InputTorque  MotionActuationMode=ComputedMotion  SensePosition=on  SenseVelocity=on  SenseAcceleration=off  SenseTorqueForce=off  SenseLowerLimitTorqueForce=off  SenseUpperLimitTorqueForce=off  LowerLimitSpecify=on  LowerLimitBound=-9.25  LowerLimitBoundUnits=m  LowerLimitStiffness=1e6  LowerLimitStiffnessUnits=N/m  LowerLimitDamping=1e3  LowerLimitDampingUnits=N/(m/s)  LowerLimitTransitionRegionWidth=1e-4  LowerLimitTransitionRegionWidthUnits=m  UpperLimitSpecify=on  UpperLimitBound=9.25  UpperLimitBoundUnits=m  UpperLimitStiffness=1e6  UpperLimitStiffnessUnits=N/m  UpperLimitDamping=1e3  UpperLimitDampingUnits=N/(m/s)  UpperLimitTransitionRegionWidth=1e-4  UpperLimitTransitionRegionWidthUnits=m  PositionTargetSpecify=off  PositionTargetPriority=High  PositionTargetValue=0  PositionTargetValueUnits=m  VelocityTargetSpecify=off  VelocityTargetPriority=High  VelocityTargetValue=0  VelocityTargetValueUnits=m/s
  Revolute Joint : sm_lib/Joints/Revolute Joint  JointMode=Normal  SenseConstraintForce=off  SenseConstraintForceX=off  SenseConstraintForceY=off  SenseConstraintForceZ=off  SenseConstraintTorque=off  SenseConstraintTorqueX=off  SenseConstraintTorqueY=off  SenseConstraintTorqueZ=off  SenseTotalForce=off  SenseTotalForceX=off  SenseTotalForceY=off  SenseTotalForceZ=off  SenseTotalTorque=off  SenseTotalTorqueX=off  SenseTotalTorqueY=off  SenseTotalTorqueZ=off  CompositeWrenchDir=FollowerOnBase  CompositeWrenchFrame=BaseFrame  EquilibriumPosition=0  EquilibriumPositionUnits=deg  SpringStiffness=0  SpringStiffnessUnits=N*m/deg  DampingCoefficient=F1  DampingCoefficientUnits=N*m/(deg/s)  TorqueActuationMode=InputTorque  MotionActuationMode=ComputedMotion  SensePosition=on  SenseVelocity=on  SenseAcceleration=off  SenseTorqueForce=off  SenseLowerLimitTorqueForce=off  SenseUpperLimitTorqueForce=off  LowerLimitSpecify=off  LowerLimitBound=-90  LowerLimitBoundUnits=deg  LowerLimitStiffness=1e4  LowerLimitStiffnessUnits=N*m/deg  LowerLimitDamping=10  LowerLimitDampingUnits=N*m/(deg/s)  LowerLimitTransitionRegionWidth=0.1  LowerLimitTransitionRegionWidthUnits=deg  UpperLimitSpecify=off  UpperLimitBound=90  UpperLimitBoundUnits=deg  UpperLimitStiffness=1e4  UpperLimitStiffnessUnits=N*m/deg  UpperLimitDamping=10  UpperLimitDampingUnits=N*m/(deg/s)  UpperLimitTransitionRegionWidth=0.1  UpperLimitTransitionRegionWidthUnits=deg  PositionTargetSpecify=off  PositionTargetPriority=Low  PositionTargetValue=0.001  PositionTargetValueUnits=deg  VelocityTargetSpecify=off  VelocityTargetPriority=High  VelocityTargetValue=0  VelocityTargetValueUnits=deg/s
  Revolute Joint1 : sm_lib/Joints/Revolute Joint  JointMode=Normal  SenseConstraintForce=off  SenseConstraintForceX=off  SenseConstraintForceY=off  SenseConstraintForceZ=off  SenseConstraintTorque=off  SenseConstraintTorqueX=off  SenseConstraintTorqueY=off  SenseConstraintTorqueZ=off  SenseTotalForce=off  SenseTotalForceX=off  SenseTotalForceY=off  SenseTotalForceZ=off  SenseTotalTorque=off  SenseTotalTorqueX=off  SenseTotalTorqueY=off  SenseTotalTorqueZ=off  CompositeWrenchDir=FollowerOnBase  CompositeWrenchFrame=BaseFrame  EquilibriumPosition=0  EquilibriumPositionUnits=deg  SpringStiffness=0  SpringStiffnessUnits=N*m/deg  DampingCoefficient=F2  DampingCoefficientUnits=N*m/(deg/s)  TorqueActuationMode=InputTorque  MotionActuationMode=ComputedMotion  SensePosition=on  SenseVelocity=on  SenseAcceleration=off  SenseTorqueForce=off  SenseLowerLimitTorqueForce=off  SenseUpperLimitTorqueForce=off  LowerLimitSpecify=off  LowerLimitBound=-90  LowerLimitBoundUnits=deg  LowerLimitStiffness=1e4  LowerLimitStiffnessUnits=N*m/deg  LowerLimitDamping=10  LowerLimitDampingUnits=N*m/(deg/s)  LowerLimitTransitionRegionWidth=0.1  LowerLimitTransitionRegionWidthUnits=deg  UpperLimitSpecify=off  UpperLimitBound=90  UpperLimitBoundUnits=deg  UpperLimitStiffness=1e4  UpperLimitStiffnessUnits=N*m/deg  UpperLimitDamping=10  UpperLimitDampingUnits=N*m/(deg/s)  UpperLimitTransitionRegionWidth=0.1  UpperLimitTransitionRegionWidthUnits=deg  PositionTargetSpecify=off  PositionTargetPriority=Low  PositionTargetValue=0.001  PositionTargetValueUnits=deg  VelocityTargetSpecify=off  VelocityTargetPriority=High  VelocityTargetValue=0  VelocityTargetValueUnits=deg/s
  Rigid Transform1 : sm_lib/Frames and Transforms/Rigid Transform  TranslationMethod=StandardAxis  TranslationStandardOffset=0  TranslationLengthUnit=m  TranslationStandardAxis=+X  TranslationCartesianOffset=[0 0 0]  TranslationROffset=0  TranslationROffsetUnits=m  TranslationZOffset=0  TranslationZOffsetUnits=m  TranslationThetaOffset=0  TranslationThetaOffsetUnits=deg  RotationMethod=RotationSequence  RotationAngleUnits=deg  RotationStandardAxis=+Z  RotationAngle=0.0  RotationArbitraryAxis=[0 0 1]  FollAlignAxisA=+X  BaseAlignAxisA=+Y  FollAlignAxisB=+Y  BaseAlignAxisB=+Z  RotationSequenceAxes=FollowerAxes  RotationSequence=XYZ  RotationSequenceAngles=[270 0 0]  RotationSequenceAnglesUnits=deg  RotationMatrix=[1 0 0; 0 1 0; 0 0 1]
  Rigid Transform2 : sm_lib/Frames and Transforms/Rigid Transform  TranslationMethod=StandardAxis  TranslationStandardOffset=barra1_long  TranslationLengthUnit=m  TranslationStandardAxis=-X  TranslationCartesianOffset=[0 0 0]  TranslationROffset=0  TranslationROffsetUnits=m  TranslationZOffset=0  TranslationZOffsetUnits=m  TranslationThetaOffset=0  TranslationThetaOffsetUnits=deg  RotationMethod=RotationSequence  RotationAngleUnits=deg  RotationStandardAxis=+Z  RotationAngle=0.0  RotationArbitraryAxis=[0 0 1]  FollAlignAxisA=+X  BaseAlignAxisA=+Y  FollAlignAxisB=+Y  BaseAlignAxisB=+Z  RotationSequenceAxes=FollowerAxes  RotationSequence=XYZ  RotationSequenceAngles=[0 0 0]  RotationSequenceAnglesUnits=deg  RotationMatrix=[1 0 0; 0 1 0; 0 0 1]
  Rigid Transform4 : sm_lib/Frames and Transforms/Rigid Transform  TranslationMethod=StandardAxis  TranslationStandardOffset=0  TranslationLengthUnit=m  TranslationStandardAxis=+Z  TranslationCartesianOffset=[0 0 0]  TranslationROffset=0  TranslationROffsetUnits=m  TranslationZOffset=0  TranslationZOffsetUnits=m  TranslationThetaOffset=0  TranslationThetaOffsetUnits=deg  RotationMethod=RotationSequence  RotationAngleUnits=deg  RotationStandardAxis=+Z  RotationAngle=0.0  RotationArbitraryAxis=[0 0 1]  FollAlignAxisA=+X  BaseAlignAxisA=+Y  FollAlignAxisB=+Y  BaseAlignAxisB=+Z  RotationSequenceAxes=FollowerAxes  RotationSequence=XYZ  RotationSequenceAngles=[0 0 0]  RotationSequenceAnglesUnits=deg  RotationMatrix=[1 0 0; 0 1 0; 0 0 1]
  Simulink-PS Converter : nesl_utility/Simulink-PS Converter  PhysicalDomain=network_engine_domain  SubClassName=ps_input  LeftPortType=input  RightPortType=output  PseudoPeriodic=off  Frequencies=[]  NoiseDistribution=none  NoiseParameters=[]  Unit=1  AffineConversion=off  FilteringAndDerivatives=provide  SimscapeFilterOrder=1  InputFilterTimeConstant=0.001  UdotUserProvided=0
      settings: SourceProductBaseCode=PW,SS
  Simulink-PS Converter1 : nesl_utility/Simulink-PS Converter  PhysicalDomain=network_engine_domain  SubClassName=ps_input  LeftPortType=input  RightPortType=output  PseudoPeriodic=off  Frequencies=[]  NoiseDistribution=none  NoiseParameters=[]  Unit=1  AffineConversion=off  FilteringAndDerivatives=provide  SimscapeFilterOrder=1  InputFilterTimeConstant=0.001  UdotUserProvided=0
      settings: SourceProductBaseCode=PW,SS
  Simulink-PS Converter2 : nesl_utility/Simulink-PS Converter  PhysicalDomain=network_engine_domain  SubClassName=ps_input  LeftPortType=input  RightPortType=output  PseudoPeriodic=off  Frequencies=[]  NoiseDistribution=none  NoiseParameters=[]  Unit=1  AffineConversion=off  FilteringAndDerivatives=provide  SimscapeFilterOrder=1  InputFilterTimeConstant=0.001  UdotUserProvided=0
      settings: SourceProductBaseCode=PW,SS
  Solver Configuration : nesl_utility/Solver Configuration  PhysicalDomain=network_engine_domain  SubClassName=solver  LeftPortType=input  RightPortType=generic  Tones=[]  Harmonics=[]  SimulateNoise=off  Profile=off  UseLocalSampling=off  EnableSwitchedLinearOptims=on  FrequencyDomain=off  UseCCode=off  RelTol=0.001  AbsTol=1e-06  MinStep=1e-09  ToWorkspace=off  RevertToSquareIcSolve=off  NumHomotopyIterations=100  PhasorMode=off  PhasorModeNumHarmonics=1  DoDC=off  ResidualTolerance=1e-09  UseLocalSolver=off  LocalSolverChoice=NE_BACKWARD_EULER_ADVANCER  LocalSolverSampleTime=0.001  DoFixedCost=off  MaxNonlinIter=3  MaxModeIter=2  ComputeImpulses=off  ImpulseIterations=2  LinearAlgebra=auto  EquationFormulation=NE_TIME_EF  DelaysMemoryBudget=1024  AutomaticFiltering=on  FilteringTimeConstant=0.001  PartitionStorageMethod=AS_NEEDED  PartitionMemoryBudget=1024  PartitionMethod=ROBUST
      settings: SourceProductBaseCode=PW,SS
  World Frame : sm_lib/Frames and Transforms/World Frame
  p : Outport
  v : Outport  Port=2
  q1 : Outport  Port=3
  w1 : Outport  Port=4
  q2 : Outport  Port=5
  w2 : Outport  Port=6
  wires:
  PS-Simulink Converter/1 -> [p]
  PS-Simulink Converter3/1 -> [q1]
  [q1] -> q1/1
  [p] -> p/1
  PS-Simulink Converter1/1 -> [v]
  PS-Simulink Converter2/1 -> [w1]
  [w1] -> w1/1
  [v] -> v/1
  u1/1 -> Simulink-PS Converter/1
  PS-Simulink Converter5/1 -> [q2]
  PS-Simulink Converter4/1 -> [w2]
  [w2] -> w2/1
  [q2] -> q2/1
  u2/1 -> Simulink-PS Converter1/1
  u3/1 -> Simulink-PS Converter2/1
  connections:
  PS-Simulink Converter1/LConn1 -- Prismatic Joint/RConn3
  Bar1/LConn1 -- Rigid Transform4/RConn1 -- Rigid Transform2/LConn1
  Rigid Transform4/LConn1 -- Revolute Joint/RConn1
  Base/RConn1 -- Config/RConn1 -- Solver Configuration/RConn1 -- World Frame/RConn1 -- Cart Transform/LConn1 -- Base/RConn3 -- Base/RConn2
  Cart Transform/RConn1 -- Prismatic Joint/LConn1
  PS-Simulink Converter/LConn1 -- Prismatic Joint/RConn2
  Simulink-PS Converter/RConn1 -- Prismatic Joint/LConn2
  PS-Simulink Converter2/LConn1 -- Revolute Joint/RConn3
  Rigid Transform1/RConn1 -- Revolute Joint/LConn1
  Revolute Joint/RConn2 -- PS-Simulink Converter3/LConn1
  Rigid Transform1/LConn1 -- Prismatic Joint/RConn1 -- Carro/RConn1
  PS-Simulink Converter4/LConn1 -- Revolute Joint1/RConn3
  PS-Simulink Converter5/LConn1 -- Revolute Joint1/RConn2
  Revolute Joint1/RConn1 -- Bar2/LConn1
  Rigid Transform2/RConn1 -- Revolute Joint1/LConn1
  Simulink-PS Converter1/RConn1 -- Revolute Joint/LConn2
  Simulink-PS Converter2/RConn1 -- Revolute Joint1/LConn2

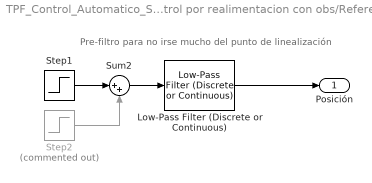
== system TPF_Control_Automatico_SLX/Control por realimentacion con obs/Referencia ==
  note: Pre-filtro para no irse mucho del punto de linealización
  Low-Pass Filter (Discrete or Continuous) : eeGeneralControl/Low-Pass Filter (Discrete or Continuous)  K=1  T=1  B=inf  A=-inf  init_option=Inherited from block input  x0=0  Ts=-1
  Step1 : Step  After=4  SampleTime=0
  Step2 : Step  Commented=on  Time=8  After=-8  SampleTime=0
  Sum2 : Sum  Inputs=|++
  Posición : Outport
  wires:
  Step2/1 -> Sum2/2
  Sum2/1 -> Low-Pass Filter (Discrete or Continuous)/1
  Low-Pass Filter (Discrete or Continuous)/1 -> Posición/1
  Step1/1 -> Sum2/1
